simulink model "sim_ex_3"  (Simulink 7.7)
settings: Solver=ode45  StartTime=0.0  StopTime=10.0  RelTol=1e-3
settings Model: Creator=cjz  LastModifiedBy=cjz

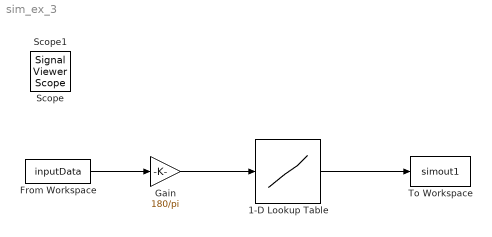
== system sim_ex_3 ==
  1-D Lookup Table : Lookup_n-D  NumberOfTableDimensions=1  BreakpointsForDimension1=[0 90]  Table=[0.5 4.5]  RndMeth=Simplest  InputSameDT=on
  From Workspace : FromWorkspace  VariableName=inputData  SampleTime=0
  Gain : Gain  Gain=180/pi
  To Workspace : ToWorkspace  VariableName=simout1  SampleTime=-1  SaveFormat=Structure
  Scope : SignalViewerScope  IOType=viewer  RefreshTime=0.035000
      settings: TimeRange=10  YMin=0  YMax=6
  Scope1 : SignalViewerScope  IOType=viewer  RefreshTime=0.035000
      settings: TimeRange=10  YMin=0  YMax=100
  wires:
  From Workspace/1 -> Gain/1
  Gain/1 -> 1-D Lookup Table/1
  1-D Lookup Table/1 -> To Workspace/1
